simulink model "KF_discreto_TEST"  (R2023b)
settings: Solver=VariableStepAuto  StartTime=0.0  StopTime=10.0  RelTol=1e-3
values from neighbouring files (symbols this model uses):
  A = [0 0 1 0 ... (first row only)    [MPC_RFJ.m]    (also in MPC_integral_RFJ.m; MPC_main_realtime.m; MPCintegral_main_realtime.m)
  B = eta_m*eta_g*Kc*Kg/Rm*B0    [MPC_RFJ.m]    (also in MPC_integral_RFJ.m; MPC_main_realtime.m; MPCintegral_main_realtime.m)
  C = [1 1 0 0 ... (first row only)    [MPC_RFJ.m]    (also in MPC_integral_RFJ.m = [1 1 0 0]; MPC_main_realtime.m = [1 0 0 0;0 1 0 0]; MPCintegral_main_realtime.m = [1 0 0 0;0 1 0 0])
  D = zeros(1,1)    [MPC_RFJ.m]    (also in MPC_integral_RFJ.m; MPC_main_realtime.m; MPCintegral_main_realtime.m)
  Ts = 0.1    [MPC_RFJ.m]    (also in MPC_integral_RFJ.m; MPC_main_realtime.m; MPCintegral_main_realtime.m)
undefined symbols (not defined in the file or in its folder): A_kf_dt, B_kf_dt, C_kf_dt, D_kf_dt, Kenl_lqr
settings Model: Creator=marco  LastModifiedBy=marco

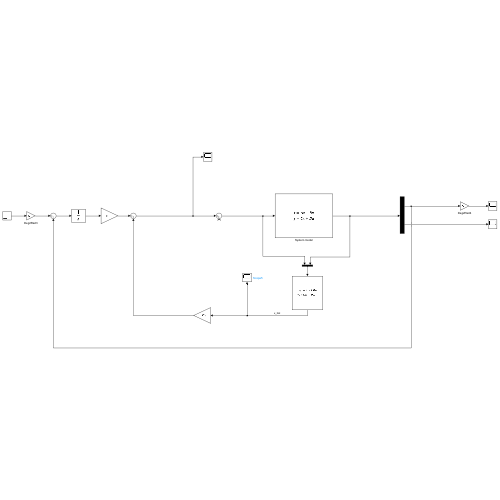
[thumbnail: Simulink's stored preview of the top-level diagram]
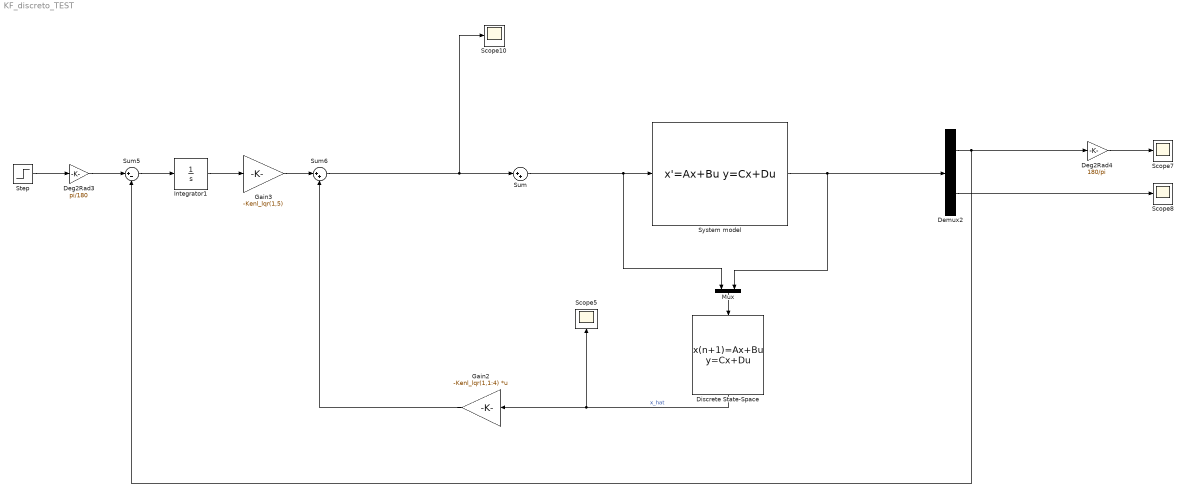
== system KF_discreto_TEST ==
  Deg2Rad3 : Gain  Gain=pi/180
  Deg2Rad4 : Gain  Gain=180/pi
  Demux2 : Demux  Outputs=2
  Discrete State-Space : DiscreteStateSpace  A=A_kf_dt  B=B_kf_dt  C=C_kf_dt  D=D_kf_dt  SampleTime=Ts
  Gain2 : Gain  Gain=-Kenl_lqr(1,1:4)  Multiplication=Matrix(K*u)
  Gain3 : Gain  Gain=-Kenl_lqr(1,5)
  Integrator1 : Integrator
  Mux : Mux  Inputs=2
  Scope{5,7..8,10} (4 alike) : Scope
  Step : Step  After=90  SampleTime=0
  Sum : Sum  Inputs=|++
  Sum5 : Sum  Inputs=|+-
  Sum6 : Sum  Inputs=|++
  System model : StateSpace  A=A  B=B  C=C  D=D  InitialCondition=[0 0 0 0]
  wires:
  Sum/1 -> Mux/1, System model/1
  Gain3/1 -> Sum6/1
  Mux/1 -> Discrete State-Space/1
  Discrete State-Space/1 -> Gain2/1, Scope5/1  "x_hat"
  Sum5/1 -> Integrator1/1
  Demux2/2 -> Scope8/1
  Gain2/1 -> Sum6/2
  Sum6/1 -> Sum/1, Scope10/1
  Deg2Rad4/1 -> Scope7/1
  Demux2/1 -> Deg2Rad4/1, Sum5/2
  Deg2Rad3/1 -> Sum5/1
  System model/1 -> Mux/2, Demux2/1
  Integrator1/1 -> Gain3/1
  Step/1 -> Deg2Rad3/1
